simulink model "bh_wheel_dynamics_model_SEME"  (R2019a)
settings: Solver=ode45  StartTime=0.0  StopTime=80  FixedStep=0.001  RelTol=1e-6  EnableMultiTasking=on
undefined symbols (not defined in the file): sigbuilder_block
libraries: simulink_extras x8
settings Model: Creator=bhorton  LastModifiedBy=bhorton
settings SolverCC: ZeroCrossAlgorithm=Adaptive
settings DataIOCC: SaveOutput=off  SignalLogging=off  DSMLogging=off  VisualizeSimOutput=off  SaveTime=off  ReturnWorkspaceOutputs=off
settings OptimizationCC: LifeSpan=inf
settings DebuggingCC: AllowSymbolicDim=off  SFUnexpectedBacktrackingDiag=warning  SFNoUnconditionalDefaultTransitionDiag=warning  SFExecutionAtInitializationDiag=none  ArithmeticOperatorsInVariantConditions=warning
settings ModelReferenceCC: PropagateSignalLabelsOutOfModel=off
settings SFSimCC: SimUseLocalCustomCode=off
settings RTWCC: RTWUseLocalCustomCode=off
settings CodeAppCC: StateflowObjectComments=on
settings GRTTargetCC: TargetLangStandard=C89/C90 (ANSI)
settings ConfigComp: CovMetricSettings=dw  CovHtmlReporting=on  CovSaveCumulativeToWorkspaceVar=on  CovSaveSingleToWorkspaceVar=on  CovExternalEMLEnable=off
settings SimscapeCC: SimscapeNormalizeSystem=off

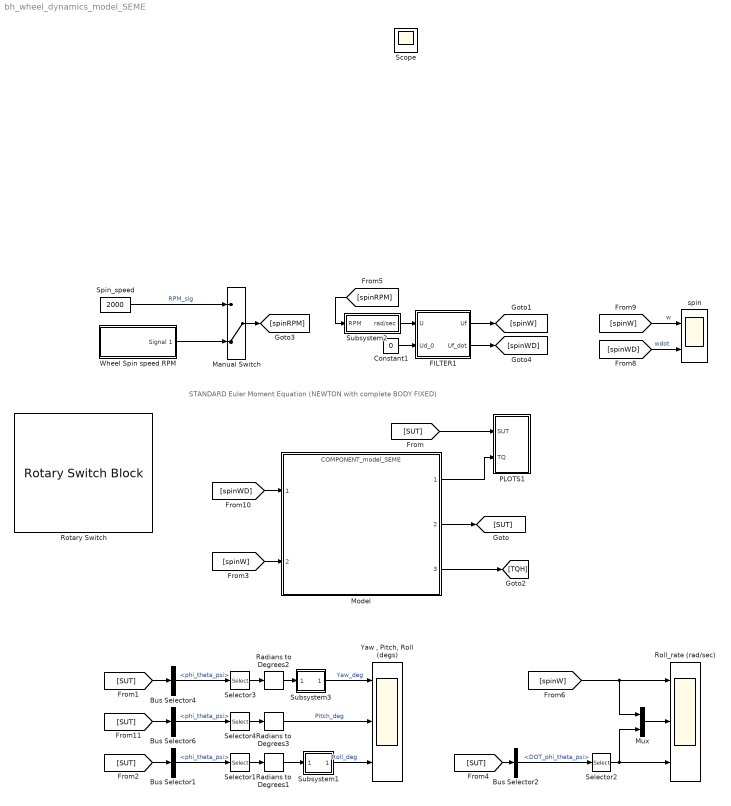
== system bh_wheel_dynamics_model_SEME ==
  note: STANDARD Euler Moment Equation (NEWTON with complete BODY FIXED)
  Bus Selector1 : BusSelector  OutputSignals=phi_theta_psi
  Bus Selector2 : BusSelector  OutputSignals=DOT_phi_theta_psi
  Bus Selector4 : BusSelector  OutputSignals=phi_theta_psi
  Bus Selector6 : BusSelector  OutputSignals=phi_theta_psi
  Constant1 : Constant  Value=0
  FILTER1 : Subsystem
  Manual Switch : ManualSwitch  CurrentSetting=0
  Model : ModelReference  ModelNameDialog=COMPONENT_model_SEME.slx  SimulationMode=Normal  ModelReferenceVersion=1.561
  Mux : Mux  Inputs=2
  PLOTS1 : Subsystem
  Radians to Degrees1 : simulink_extras/Transformations/Radians to Degrees
  Radians to Degrees2 : simulink_extras/Transformations/Radians to Degrees
  Radians to Degrees3 : simulink_extras/Transformations/Radians to Degrees
  Roll_rate (rad/sec) : Scope  NumInputPorts=3
  Rotary Switch : RotarySwitchBlock
      settings: Values={{'ZERO', '150', '500', '750', '1000', '1500', '2000'}, [0 150 500 750 1000 1500 2000]}
  Selector1 : Selector  InputPortWidth=3  IndexOptions=Index vector (dialog)  Indices=3  OutputSizes=1
  Selector2 : Selector  InputPortWidth=3  IndexOptions=Index vector (dialog)  Indices=3  OutputSizes=1
  Selector3 : Selector  InputPortWidth=3  IndexOptions=Index vector (dialog)  Indices=1  OutputSizes=1
  Selector4 : Selector  InputPortWidth=3  IndexOptions=Index vector (dialog)  Indices=2  OutputSizes=1
  Spin_speed : Constant  Value=2000
  Subsystem1 : Subsystem
      mask Display: disp(sprintf('Mod\n360'))
  Subsystem2 : Subsystem
  Subsystem3 : Subsystem
      mask Display: disp(sprintf('Mod\n360'))
  Wheel Spin speed RPM : Subsystem  Tag=STV Subsys  LoadFcn=sigbuilder_block('load');  StartFcn=sigbuilder_block('start');  StopFcn=sigbuilder_block('stop');  ClipboardFcn=sigbuilder_block('clipboard');  mask(Sigbuilder block){tuvar=[0:10]}
      mask help: Simulink:masks:SigbuilderBlock_MD
      mask init:
      | if ~strcmp(get_param(bdroot(gcbh),'SimulationStatus'),'stopped') tuvar = sigbuilder_block('maskInit'); end
      settings: CopyFcn=sigbuilder_block('copy');  DeleteFcn=sigbuilder_block('delete');  ModelCloseFcn=sigbuilder_block('modelClose');  PreSaveFcn=sigbuilder_block('preSave');  PauseFcn=sigbuilder_block('pause');  ContinueFcn=sigbuilder_block('continue');  NameChangeFcn=sigbuilder_block('namechange');  OpenFcn=sigbuilder_block('open',[6 6 1428 740.25 ]);  CloseFcn=sigbuilder_block('close');
      mask Display: plot(0, 0, 100, 100,[2, 2, 32, 32, 2], [68, 8, 8, 68, 68],[32, 2], [38, 38], [32, 19, 2],[53, 60, 44], [32, 17, 17, 2],[16, 16, 31, 31]);txt = getActiveGroup(gcbh);text(2, 100, txt,'verticalAlignment', 'top');
  "Yaw , Pitch, Roll (degs)" : Scope  NumInputPorts=3
  spin : Scope  NumInputPorts=2
  Scope : Scope
  wires:
  Spin_speed/1 -> Manual Switch/1  "RPM_sig"
  Wheel Spin speed RPM/1(Signal 1) -> Manual Switch/2
  Manual Switch/1 -> [spinRPM]
  Subsystem2/1(rad/sec) -> FILTER1/1(U)
  Constant1/1 -> FILTER1/2(Ud_0)
  [spinRPM] -> Subsystem2/1(RPM)
  FILTER1/1(Uf) -> [spinW]
  FILTER1/2(Uf_dot) -> [spinWD]
  [spinWD] -> spin/2  "wdot"
  [spinW] -> spin/1  "w"
  [spinWD] -> Model/1
  Selector4/1 -> Radians to Degrees3/1
  Selector3/1 -> Radians to Degrees2/1
  Bus Selector4/1 -> Selector3/1  "<phi_theta_psi>"
  Subsystem3/1(Out1) -> "Yaw , Pitch, Roll (degs)"/1  "Yaw_deg"
  [SUT] -> Bus Selector4/1
  Radians to Degrees3/1 -> "Yaw , Pitch, Roll (degs)"/2  "Pitch_deg"
  Radians to Degrees2/1 -> Subsystem3/1(In1)
  Bus Selector6/1 -> Selector4/1  "<phi_theta_psi>"
  [SUT] -> Bus Selector6/1
  Bus Selector1/1 -> Selector1/1  "<phi_theta_psi>"
  [SUT] -> Bus Selector1/1
  Selector1/1 -> Radians to Degrees1/1
  Radians to Degrees1/1 -> Subsystem1/1(In1)
  Subsystem1/1(Out1) -> "Yaw , Pitch, Roll (degs)"/3  "Roll_deg"
  [SUT] -> Bus Selector2/1
  Bus Selector2/1 -> Selector2/1  "<DOT_phi_theta_psi>"
  Selector2/1 -> Mux/2, Roll_rate (rad/sec)/3
  [spinW] -> Mux/1, Roll_rate (rad/sec)/1
  Mux/1 -> Roll_rate (rad/sec)/2
  Model/3 -> [TQH]
  Model/2 -> [SUT]
  Model/1 -> PLOTS1/2(TQ)
  [SUT] -> PLOTS1/1(SUT)
  [spinW] -> Model/2

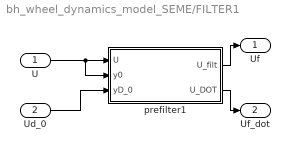
== system bh_wheel_dynamics_model_SEME/FILTER1 ==
  U : Inport
  Ud_0 : Inport  Port=2
  prefilter1 : Subsystem  mask(Derivative Estimation){wn=2*pi*5, p=1}
      mask prompts: wn "Natural frequency, wn (rad/sec)"; p "Damping ratio, p"
      mask help:
      | A simple derivative estimator using a 2nd order representation between input and output.
      |
      | The integrators use a discrete FORWARd Euler rule, and a sample time needs to be specified.
      mask init:
      | str1 = sprintf('wn = %.2f', wn);
      | str2 = sprintf('p  = %.2f', p);
      | %str3 = sprintf('dt = %.2f', dt);
      | %str = char(str1,str2,str3);
      | %str3 = sprintf('dt = %.2f', dt);
      | str = char(str1,str2);
      mask Display: disp(str)
  Uf : Outport
  Uf_dot : Outport  Port=2
  wires:
  Ud_0/1 -> prefilter1/3(yD_0)
  prefilter1/2(U_DOT) -> Uf_dot/1
  prefilter1/1(U_filt) -> Uf/1
  U/1 -> prefilter1/2(y0), prefilter1/1(U)

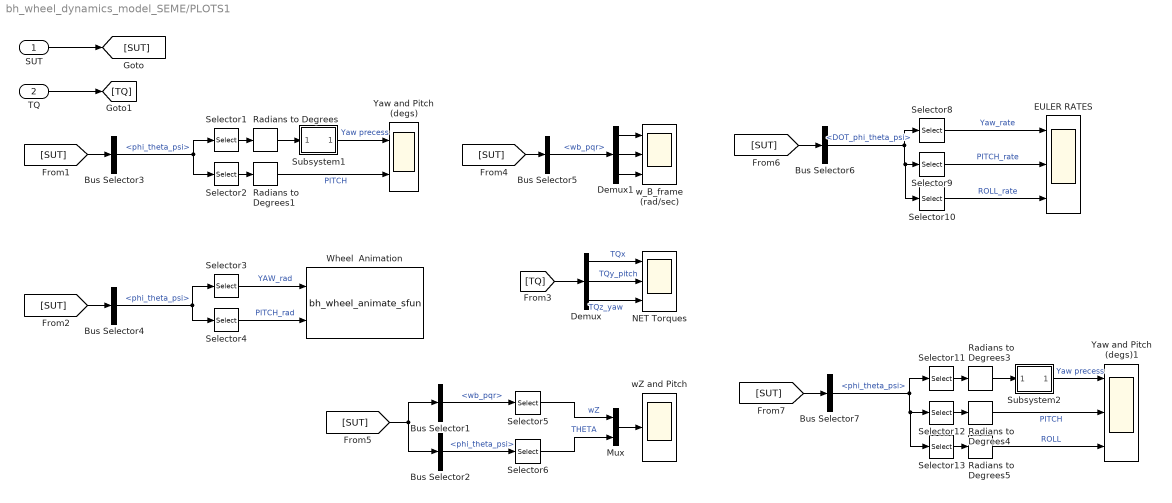
== system bh_wheel_dynamics_model_SEME/PLOTS1 ==
  SUT : Inport
  TQ : Inport  Port=2
  Bus Selector1 : BusSelector  OutputSignals=wb_pqr
  Bus Selector{2..4,7} (4 alike) : BusSelector  OutputSignals=phi_theta_psi
  Bus Selector5 : BusSelector  OutputSignals=wb_pqr
  Bus Selector6 : BusSelector  OutputSignals=DOT_phi_theta_psi
  Demux : Demux  Outputs=3
  Demux1 : Demux  Outputs=3
  EULER RATES : Scope  NumInputPorts=3
  Mux : Mux  Inputs=2
  NET Torques : Scope  NumInputPorts=3
  Radians to Degrees{,1,3..5} (5 alike) : simulink_extras/Transformations/Radians to Degrees
  Selector{1,3,8,11} (4 alike) : Selector  InputPortWidth=3  IndexOptions=Index vector (dialog)  Indices=1  OutputSizes=1
  Selector10 : Selector  InputPortWidth=3  IndexOptions=Index vector (dialog)  Indices=3  OutputSizes=1
  Selector{2,4,6,9,12} (5 alike) : Selector  InputPortWidth=3  IndexOptions=Index vector (dialog)  Indices=2  OutputSizes=1
  Selector13 : Selector  InputPortWidth=3  IndexOptions=Index vector (dialog)  Indices=3  OutputSizes=1
  Selector5 : Selector  InputPortWidth=3  IndexOptions=Index vector (dialog)  Indices=3  OutputSizes=1
  Subsystem1 : Subsystem
      mask Display: disp(sprintf('Mod\n360'))
  Subsystem2 : Subsystem
      mask Display: disp(sprintf('Mod\n360'))
  Wheel  Animation : M-S-Function  FunctionName=bh_wheel_animate_sfun  Parameters=0.1, r, d
  Yaw and Pitch (degs) : Scope  NumInputPorts=2
  Yaw and Pitch (degs)1 : Scope  NumInputPorts=3
  wZ and Pitch : Scope
  w_B_frame (rad/sec) : Scope  NumInputPorts=3
  wires:
  [SUT] -> Bus Selector3/1
  Bus Selector3/1 -> Selector2/1, Selector1/1  "<phi_theta_psi>"
  Selector1/1 -> Radians to Degrees/1
  Selector2/1 -> Radians to Degrees1/1
  Radians to Degrees1/1 -> Yaw and Pitch (degs)/2  "PITCH"
  Selector3/1 -> Wheel  Animation/1  "YAW_rad"
  Selector4/1 -> Wheel  Animation/2  "PITCH_rad"
  [SUT] -> Bus Selector4/1
  Bus Selector4/1 -> Selector4/1, Selector3/1  "<phi_theta_psi>"
  Demux/1 -> NET Torques/1  "TQx"
  Demux/3 -> NET Torques/3  "TQz_yaw"
  Demux/2 -> NET Torques/2  "TQy_pitch"
  [TQ] -> Demux/1
  [SUT] -> Bus Selector5/1
  Demux1/1 -> w_B_frame (rad/sec)/1
  Demux1/2 -> w_B_frame (rad/sec)/2
  Demux1/3 -> w_B_frame (rad/sec)/3
  Bus Selector5/1 -> Demux1/1  "<wb_pqr>"
  Radians to Degrees/1 -> Subsystem1/1(In1)
  Subsystem1/1(Out1) -> Yaw and Pitch (degs)/1  "Yaw precess"
  SUT/1 -> [SUT]
  TQ/1 -> [TQ]
  [SUT] -> Bus Selector2/1, Bus Selector1/1
  Bus Selector1/1 -> Selector5/1  "<wb_pqr>"
  Mux/1 -> wZ and Pitch/1
  Bus Selector2/1 -> Selector6/1  "<phi_theta_psi>"
  Selector5/1 -> Mux/1  "wZ"
  Selector6/1 -> Mux/2  "THETA"
  Selector9/1 -> EULER RATES/2  "PITCH_rate"
  Selector8/1 -> EULER RATES/1  "Yaw_rate"
  Selector10/1 -> EULER RATES/3  "ROLL_rate"
  [SUT] -> Bus Selector6/1
  Bus Selector6/1 -> Selector8/1, Selector10/1, Selector9/1  "<DOT_phi_theta_psi>"
  [SUT] -> Bus Selector7/1
  Bus Selector7/1 -> Selector13/1, Selector12/1, Selector11/1  "<phi_theta_psi>"
  Selector11/1 -> Radians to Degrees3/1
  Selector12/1 -> Radians to Degrees4/1
  Radians to Degrees4/1 -> Yaw and Pitch (degs)1/2  "PITCH"
  Radians to Degrees3/1 -> Subsystem2/1(In1)
  Subsystem2/1(Out1) -> Yaw and Pitch (degs)1/1  "Yaw precess"
  Selector13/1 -> Radians to Degrees5/1
  Radians to Degrees5/1 -> Yaw and Pitch (degs)1/3  "ROLL"

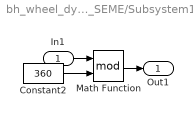
== system bh_wheel_dynamics_model_SEME/Subsystem1 ==
  In1 : Inport
  Constant2 : Constant  Value=360
  Math Function : Math  Operator=mod  SaturateOnIntegerOverflow=on
  Out1 : Outport
  wires:
  Math Function/1 -> Out1/1
  In1/1 -> Math Function/1
  Constant2/1 -> Math Function/2

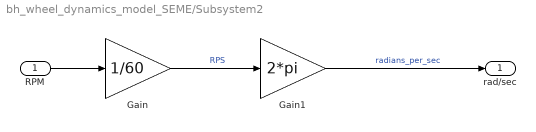
== system bh_wheel_dynamics_model_SEME/Subsystem2 ==
  RPM : Inport
  Gain : Gain  Gain=1/60
  Gain1 : Gain  Gain=2*pi
  rad/sec : Outport
  wires:
  RPM/1 -> Gain/1
  Gain/1 -> Gain1/1  "RPS"
  Gain1/1 -> rad/sec/1  "radians_per_sec"

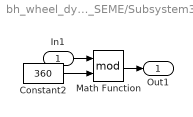
== system bh_wheel_dynamics_model_SEME/Subsystem3 ==
  In1 : Inport
  Constant2 : Constant  Value=360
  Math Function : Math  Operator=mod  SaturateOnIntegerOverflow=on
  Out1 : Outport
  wires:
  Math Function/1 -> Out1/1
  In1/1 -> Math Function/1
  Constant2/1 -> Math Function/2

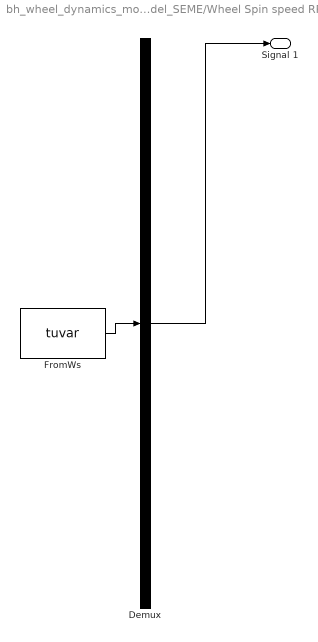
== system bh_wheel_dynamics_model_SEME/Wheel Spin speed RPM ==
  Demux : Demux  Tag=STV Demux  Outputs=1
  FromWs : FromWorkspace  Tag=STV FromWs  VariableName=tuvar  SampleTime=0
      SigBuilderData=|
      | common.afterFinalStr = 'Extrapolate'
      | common.sampleTime = 0
      | dataSet(1).timeRange = [0 60]
      | dataSet(1).name = 'RAMP_DOWN'
      | dataSet(2).timeRange = [0 80]
      | dataSet(2).name = 'STAIRCASE_DOWN'
      | dataSet(3).timeRange = [0 60]
      | dataSet(3).name = 'STAIRCASE_UP'
      | sbobj.Groups(1).Name = 'RAMP_DOWN'
      | sbobj.Groups(1).Signals.Name = 'Signal 1'
      | sbobj.Groups(1).Signals.XData = [0 60]
      | sbobj.Groups(1).Signals.YData = [2000 0]
      | sbobj.Groups(1).TimeRange = [0 60]
      | sbobj.Groups(2).Name = 'STAIRCASE_DOWN'
      | sbobj.Groups(2).Signals.Name = 'Signal 1'
      | sbobj.Groups(2).Signals.XData = [0 10.1 10.1 20 20 30 30 39.9 39.9 49.9 49.9 60.2 60.2 70 70 80]
      | sbobj.Groups(2).Signals.YData = [2000 2000 1500 1500 1000 1000 750 750 500 500 150 150 60 60 0 0]
      | sbobj.Groups(2).TimeRange = [0 80]
      | sbobj.Groups(3).Name = 'STAIRCASE_UP'
      | sbobj.Groups(3).Signals.Name = 'Signal 1'
      | sbobj.Groups(3).Signals.XData = [0 9.9 9.9 19.9 19.9 30.1 30.1 39.9 39.9 49.9 49.9 60]
      | sbobj.Groups(3).Signals.YData = [2000 2000 2200 2200 2400 2400 2610 2610 1800 1800 1600 1600]
      | sbobj.Groups(3).TimeRange = [0 60]
  Signal 1 : Outport  Tag=STV Outport
  wires:
  Demux/1 -> Signal 1/1
  FromWs/1 -> Demux/1

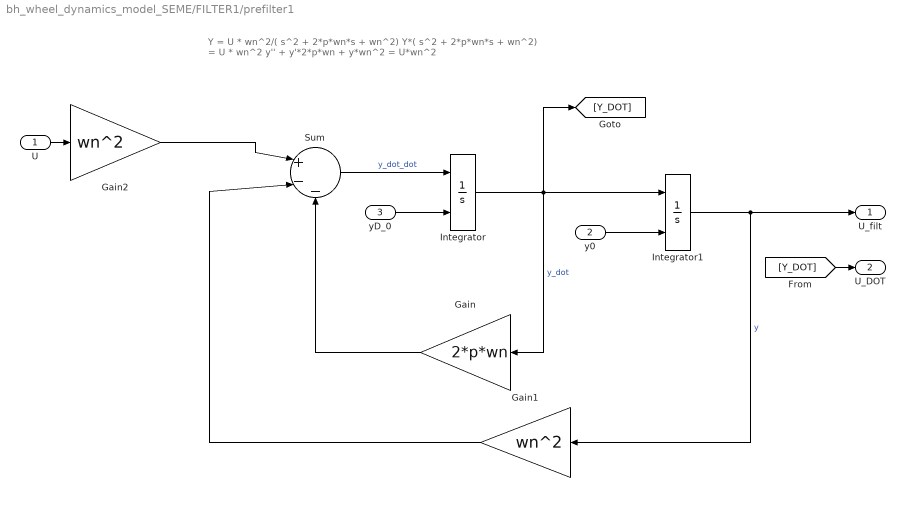
== system bh_wheel_dynamics_model_SEME/FILTER1/prefilter1 ==
  note: Y = U *     wn^2/( s^2 + 2*p*wn*s + wn^2)
      | Y*( s^2 + 2*p*wn*s + wn^2) = U * wn^2
      |
      | y'' + y'*2*p*wn + y*wn^2 = U*wn^2
  U : Inport
  y0 : Inport  Port=2
  yD_0 : Inport  Port=3
  Gain : Gain  Gain=2*p*wn
  Gain1 : Gain  Gain=wn^2
  Gain2 : Gain  Gain=wn^2
  Integrator : Integrator  InitialConditionSource=external
  Integrator1 : Integrator  InitialConditionSource=external
  Sum : Sum  Inputs=|+--
  U_filt : Outport
  U_DOT : Outport  Port=2
  wires:
  Integrator/1 -> [Y_DOT], Gain/1, Integrator1/1  "y_dot"
  Sum/1 -> Integrator/1  "y_dot_dot"
  Integrator1/1 -> Gain1/1, U_filt/1  "y"
  U/1 -> Gain2/1
  Gain2/1 -> Sum/1
  Gain/1 -> Sum/3
  Gain1/1 -> Sum/2
  [Y_DOT] -> U_DOT/1
  yD_0/1 -> Integrator/2
  y0/1 -> Integrator1/2

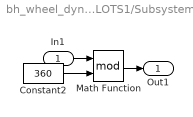
== system bh_wheel_dynamics_model_SEME/PLOTS1/Subsystem1 ==
  In1 : Inport
  Constant2 : Constant  Value=360
  Math Function : Math  Operator=mod  SaturateOnIntegerOverflow=on
  Out1 : Outport
  wires:
  Math Function/1 -> Out1/1
  In1/1 -> Math Function/1
  Constant2/1 -> Math Function/2

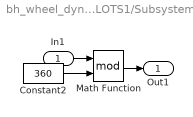
== system bh_wheel_dynamics_model_SEME/PLOTS1/Subsystem2 ==
  In1 : Inport
  Constant2 : Constant  Value=360
  Math Function : Math  Operator=mod  SaturateOnIntegerOverflow=on
  Out1 : Outport
  wires:
  Math Function/1 -> Out1/1
  In1/1 -> Math Function/1
  Constant2/1 -> Math Function/2
